simulink model "ThomBBa_Drone"  (R2023a)
settings: Solver=VariableStepAuto  StartTime=0.0  StopTime=10  RelTol=1e-3
values from neighbouring files (symbols this model uses):
  J = [0.00031              0              -0.000004657 ... (first row only)    [paramm.m]
  K = 1256.637    [paramm.m]
  Km = 6.1028207267564559047121275317652e-7    (= 6.10282072676e-07)    [paramm.m]
  Kn = 6.1028207267564559047121275317652e-7    (= 6.10282072676e-07)    [paramm.m]
  l = 0.1125    [paramm.m]
  Phi_air_damping_constant = 0    [paramm.m]
  Psi_air_damping_constant = 0    [paramm.m]
  Tau = 0.001    [paramm.m]
  Theta_air_damping_constant = 0    [paramm.m]
undefined symbols (not defined in the file or in its folder): x_air_damping_ratio, y_air_damping_ratio, z_air_damping_ratio
libraries: dspsigops x15, slpidlib x6
(part 1 of 2)
settings Model: PacingRate=1000  Creator=ThomBBa  LastModifiedBy=ThomBBa
settings DebuggingCC: AlgebraicLoopMsg=none

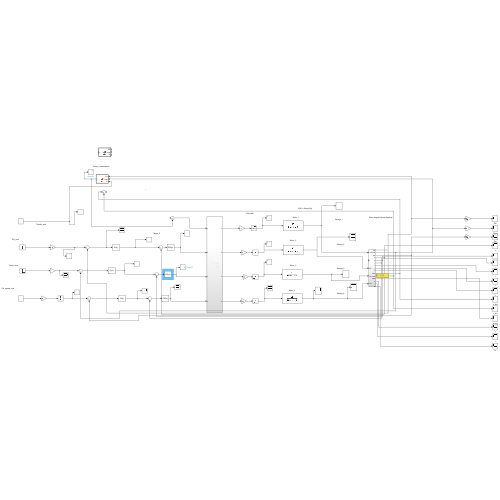
[thumbnail: Simulink's stored preview of the top-level diagram]
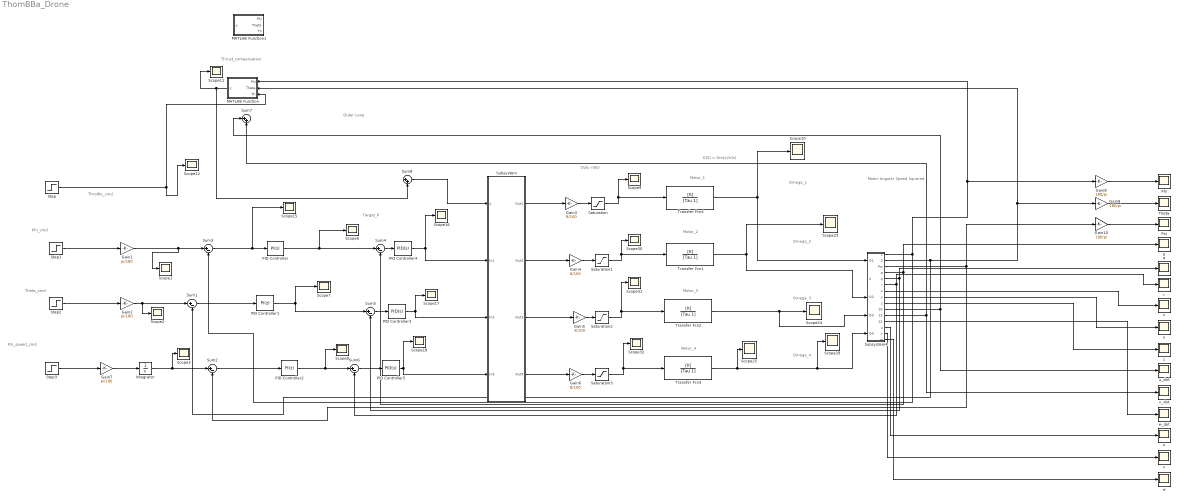
== system ThomBBa_Drone ==
  note: Thrust_compensation
  note: G(S) = Om(s)/V(s)
  note: Omega_1
  note: Motor_1
  note: Motor_2
  note: Omega_2
  note: Throttle_cmd
  note: Target_P
  note: Duty ratio
  note: Motor Angular Speed Squared
  note: Outer Loop
  note: Motor_3
  note: Motor_4
  note: Omega_4
  note: Phi_cmd
  note: Theta_cmd
  note: Psi_speed_cmd
  note: Omega_3
  Gain1 : Gain  Gain=pi/180
  Gain10 : Gain  Gain=180/pi
  Gain2 : Gain  Gain=pi/180
  Gain{3..6} (4 alike) : Gain  Gain=8/100
  Gain7 : Gain  Gain=pi/180
  Gain8 : Gain  Gain=180/pi
  Gain9 : Gain  Gain=180/pi
  Integrator : Integrator
  MATLAB Function : MATLAB Function  TreatAsAtomicUnit=on
  MATLAB Function1 : MATLAB Function  TreatAsAtomicUnit=on
  PID Controller : slpidlib/PID Controller  Controller=PI  Form=Parallel  TimeDomain=Continuous-time  UseExternalTs=off  SampleTime=-1  IntegratorMethod=Forward Euler  FilterMethod=Forward Euler  ControllerParametersSource=internal  P=3  I=0  UseKiTs=off  D=0  N=100  UseFilter=on  TunerSelectOption=Transfer Function Based (PID Tuner App)  InitialConditionSource=internal  InitialConditionForIntegrator=0  InitialConditionForFilter=0  DifferentiatorICPrevScaledInput=0  ExternalReset=none  TrackingMode=off  Kt=1  LimitOutput=off  SatLimitsSource=internal  UpperSaturationLimit=inf  LowerSaturationLimit=-inf  LinearizeAsGain=on  AntiWindupMode=none  Kb=1  LimitIntegrator=off  UpperIntegratorSaturationLimit=inf  LowerIntegratorSaturationLimit=-inf  POutMin=[]  POutMax=[]  IOutMin=[]  IOutMax=[]  DOutMin=[]  DOutMax=[]  NOutMin=[]  NOutMax=[]  SumOutMin=[]  SumOutMax=[]  SaturationOutMin=[]  SaturationOutMax=[]  PParamMin=[]  PParamMax=[]  IParamMin=[]  IParamMax=[]  DParamMin=[]  DParamMax=[]  NParamMin=[]  NParamMax=[]  KbParamMin=[]  KbParamMax=[]  KtParamMin=[]  KtParamMax=[]  KbOutMin=[]  KbOutMax=[]  KtOutMin=[]  KtOutMax=[]  IntegratorOutMin=[]  IntegratorOutMax=[]  FilterOutMin=[]  FilterOutMax=[]  SumI1OutMin=[]  SumI1OutMax=[]  SumI2OutMin=[]  SumI2OutMax=[]  SumI3OutMin=[]  SumI3OutMax=[]  SumI4OutMin=[]  SumI4OutMax=[]  SumDOutMin=[]  SumDOutMax=[]  DifferentiatorOutMin=[]  DifferentiatorOutMax=[]  FilterDiffOutCoefMin=[]  FilterDiffOutCoefMax=[]  ReciprocalOutMin=[]  ReciprocalOutMax=[]  SumDenOutMin=[]  SumDenOutMax=[]  SumNumOutMin=[]  SumNumOutMax=[]  DivideOutMin=[]  DivideOutMax=[]  UdiffTsProdOutMin=[]  UdiffTsProdOutMax=[]  NTsProdOutMin=[]  NTsProdOutMax=[]  UintegralTsProdOutMin=[]  UintegralTsProdOutMax=[]  UngainTsProdOutMin=[]  UngainTsProdOutMax=[]  ClampingZeroOutDataTypeStr=Inherit: Inherit via back propagation  ClampingZeroOutMin=[]  ClampingZeroOutMax=[]  FilterDenConstantOutDataTypeStr=Inherit: Inherit via back propagation  FilterDenConstantOutMin=[]  FilterDenConstantOutMax=[]  PCopyOutDataTypeStr=Inherit: Inherit via back propagation  PCopyOutMin=[]  PCopyOutMax=[]  NCopyOutDataTypeStr=Inherit: Inherit via back propagation  NCopyOutMin=[]  NCopyOutMax=[]  IntegratorContinuousStateAttributes=''  IntegratorStateMustResolveToSignalObject=off  IntegratorRTWStateStorageClass=Auto  FilterContinuousStateAttributes=''  FilterStateMustResolveToSignalObject=off  FilterRTWStateStorageClass=Auto  ParallelPVariant=InternalParameters  IdealPVariant=Disabled  IVariant=InternalParameters  DVariant=Disabled  IntegratorVariant=Continuous  SatVariant=Disabled  AWVariant=Passthrough  PCopyVariant=Disabled  TRVariant=Disabled  FdbkBlocksVariant=Forward  IdealPFdbkVariant=Disabled  SatFdbkVariant=Disabled  DerivativeFilterVariant=Disabled  NVariant=Disabled  NCopyVariant=Disabled_SignalSpec  FilterICVariant=Disabled  IntegratorICVariant=InternalICs  ExternalResetVariant=Disabled  TRSumVariant=Passthrough  SumFdbkVariant=Disabled  SumVariant=Sum_PI  TsampFilterVariant=InternalTs  TsampNgainVariant=Passthrough  TsampIntegralVariant=Disabled_SignalSpec  ExternalSaturationOutDataTypeStr=Inherit: Same as second input
  PID Controller1 : slpidlib/PID Controller  Controller=PI  Form=Parallel  TimeDomain=Discrete-time  UseExternalTs=off  SampleTime=-1  IntegratorMethod=Forward Euler  FilterMethod=Forward Euler  ControllerParametersSource=internal  P=3  I=0  UseKiTs=off  D=0  N=100  UseFilter=on  TunerSelectOption=Transfer Function Based (PID Tuner App)  InitialConditionSource=internal  InitialConditionForIntegrator=0  InitialConditionForFilter=0  DifferentiatorICPrevScaledInput=0  ExternalReset=none  TrackingMode=off  Kt=1  LimitOutput=off  SatLimitsSource=internal  UpperSaturationLimit=inf  LowerSaturationLimit=-inf  LinearizeAsGain=on  AntiWindupMode=none  Kb=1  LimitIntegrator=off  UpperIntegratorSaturationLimit=inf  LowerIntegratorSaturationLimit=-inf  POutMin=[]  POutMax=[]  IOutMin=[]  IOutMax=[]  DOutMin=[]  DOutMax=[]  NOutMin=[]  NOutMax=[]  SumOutMin=[]  SumOutMax=[]  SaturationOutMin=[]  SaturationOutMax=[]  PParamMin=[]  PParamMax=[]  IParamMin=[]  IParamMax=[]  DParamMin=[]  DParamMax=[]  NParamMin=[]  NParamMax=[]  KbParamMin=[]  KbParamMax=[]  KtParamMin=[]  KtParamMax=[]  KbOutMin=[]  KbOutMax=[]  KtOutMin=[]  KtOutMax=[]  IntegratorOutMin=[]  IntegratorOutMax=[]  FilterOutMin=[]  FilterOutMax=[]  SumI1OutMin=[]  SumI1OutMax=[]  SumI2OutMin=[]  SumI2OutMax=[]  SumI3OutMin=[]  SumI3OutMax=[]  SumI4OutMin=[]  SumI4OutMax=[]  SumDOutMin=[]  SumDOutMax=[]  DifferentiatorOutMin=[]  DifferentiatorOutMax=[]  FilterDiffOutCoefMin=[]  FilterDiffOutCoefMax=[]  ReciprocalOutMin=[]  ReciprocalOutMax=[]  SumDenOutMin=[]  SumDenOutMax=[]  SumNumOutMin=[]  SumNumOutMax=[]  DivideOutMin=[]  DivideOutMax=[]  UdiffTsProdOutMin=[]  UdiffTsProdOutMax=[]  NTsProdOutMin=[]  NTsProdOutMax=[]  UintegralTsProdOutMin=[]  UintegralTsProdOutMax=[]  UngainTsProdOutMin=[]  UngainTsProdOutMax=[]  ClampingZeroOutDataTypeStr=Inherit: Inherit via back propagation  ClampingZeroOutMin=[]  ClampingZeroOutMax=[]  FilterDenConstantOutDataTypeStr=Inherit: Inherit via back propagation  FilterDenConstantOutMin=[]  FilterDenConstantOutMax=[]  PCopyOutDataTypeStr=Inherit: Inherit via back propagation  PCopyOutMin=[]  PCopyOutMax=[]  NCopyOutDataTypeStr=Inherit: Inherit via back propagation  NCopyOutMin=[]  NCopyOutMax=[]  IntegratorContinuousStateAttributes=''  IntegratorStateMustResolveToSignalObject=off  IntegratorRTWStateStorageClass=Auto  FilterContinuousStateAttributes=''  FilterStateMustResolveToSignalObject=off  FilterRTWStateStorageClass=Auto  ParallelPVariant=InternalParameters  IdealPVariant=Disabled  IVariant=InternalParameters  DVariant=Disabled  IntegratorVariant=Discrete  SatVariant=Disabled  AWVariant=Passthrough  PCopyVariant=Disabled  TRVariant=Disabled  FdbkBlocksVariant=Forward  IdealPFdbkVariant=Disabled  SatFdbkVariant=Disabled  DerivativeFilterVariant=Disabled  NVariant=Disabled  NCopyVariant=Disabled_SignalSpec  FilterICVariant=Disabled  IntegratorICVariant=InternalICs  ExternalResetVariant=Disabled  TRSumVariant=Passthrough  SumFdbkVariant=Disabled  SumVariant=Sum_PI  TsampFilterVariant=InternalTs  TsampNgainVariant=Passthrough  TsampIntegralVariant=Disabled_SignalSpec  ExternalSaturationOutDataTypeStr=Inherit: Same as second input
  PID Controller2 : slpidlib/PID Controller  Controller=PI  Form=Parallel  TimeDomain=Discrete-time  UseExternalTs=off  SampleTime=-1  IntegratorMethod=Forward Euler  FilterMethod=Forward Euler  ControllerParametersSource=internal  P=1  I=0  UseKiTs=off  D=0  N=100  UseFilter=on  TunerSelectOption=Transfer Function Based (PID Tuner App)  InitialConditionSource=internal  InitialConditionForIntegrator=0  InitialConditionForFilter=0  DifferentiatorICPrevScaledInput=0  ExternalReset=none  TrackingMode=off  Kt=1  LimitOutput=off  SatLimitsSource=internal  UpperSaturationLimit=inf  LowerSaturationLimit=-inf  LinearizeAsGain=on  AntiWindupMode=none  Kb=1  LimitIntegrator=off  UpperIntegratorSaturationLimit=inf  LowerIntegratorSaturationLimit=-inf  POutMin=[]  POutMax=[]  IOutMin=[]  IOutMax=[]  DOutMin=[]  DOutMax=[]  NOutMin=[]  NOutMax=[]  SumOutMin=[]  SumOutMax=[]  SaturationOutMin=[]  SaturationOutMax=[]  PParamMin=[]  PParamMax=[]  IParamMin=[]  IParamMax=[]  DParamMin=[]  DParamMax=[]  NParamMin=[]  NParamMax=[]  KbParamMin=[]  KbParamMax=[]  KtParamMin=[]  KtParamMax=[]  KbOutMin=[]  KbOutMax=[]  KtOutMin=[]  KtOutMax=[]  IntegratorOutMin=[]  IntegratorOutMax=[]  FilterOutMin=[]  FilterOutMax=[]  SumI1OutMin=[]  SumI1OutMax=[]  SumI2OutMin=[]  SumI2OutMax=[]  SumI3OutMin=[]  SumI3OutMax=[]  SumI4OutMin=[]  SumI4OutMax=[]  SumDOutMin=[]  SumDOutMax=[]  DifferentiatorOutMin=[]  DifferentiatorOutMax=[]  FilterDiffOutCoefMin=[]  FilterDiffOutCoefMax=[]  ReciprocalOutMin=[]  ReciprocalOutMax=[]  SumDenOutMin=[]  SumDenOutMax=[]  SumNumOutMin=[]  SumNumOutMax=[]  DivideOutMin=[]  DivideOutMax=[]  UdiffTsProdOutMin=[]  UdiffTsProdOutMax=[]  NTsProdOutMin=[]  NTsProdOutMax=[]  UintegralTsProdOutMin=[]  UintegralTsProdOutMax=[]  UngainTsProdOutMin=[]  UngainTsProdOutMax=[]  ClampingZeroOutDataTypeStr=Inherit: Inherit via back propagation  ClampingZeroOutMin=[]  ClampingZeroOutMax=[]  FilterDenConstantOutDataTypeStr=Inherit: Inherit via back propagation  FilterDenConstantOutMin=[]  FilterDenConstantOutMax=[]  PCopyOutDataTypeStr=Inherit: Inherit via back propagation  PCopyOutMin=[]  PCopyOutMax=[]  NCopyOutDataTypeStr=Inherit: Inherit via back propagation  NCopyOutMin=[]  NCopyOutMax=[]  IntegratorContinuousStateAttributes=''  IntegratorStateMustResolveToSignalObject=off  IntegratorRTWStateStorageClass=Auto  FilterContinuousStateAttributes=''  FilterStateMustResolveToSignalObject=off  FilterRTWStateStorageClass=Auto  ParallelPVariant=InternalParameters  IdealPVariant=Disabled  IVariant=InternalParameters  DVariant=Disabled  IntegratorVariant=Discrete  SatVariant=Disabled  AWVariant=Passthrough  PCopyVariant=Disabled  TRVariant=Disabled  FdbkBlocksVariant=Forward  IdealPFdbkVariant=Disabled  SatFdbkVariant=Disabled  DerivativeFilterVariant=Disabled  NVariant=Disabled  NCopyVariant=Disabled_SignalSpec  FilterICVariant=Disabled  IntegratorICVariant=InternalICs  ExternalResetVariant=Disabled  TRSumVariant=Passthrough  SumFdbkVariant=Disabled  SumVariant=Sum_PI  TsampFilterVariant=InternalTs  TsampNgainVariant=Passthrough  TsampIntegralVariant=Disabled_SignalSpec  ExternalSaturationOutDataTypeStr=Inherit: Same as second input
  PID Controller3 : slpidlib/PID Controller  Controller=PID  Form=Parallel  TimeDomain=Continuous-time  UseExternalTs=off  SampleTime=-1  IntegratorMethod=Forward Euler  FilterMethod=Forward Euler  ControllerParametersSource=internal  P=15  I=0  UseKiTs=off  D=3  N=100  UseFilter=on  TunerSelectOption=Transfer Function Based (PID Tuner App)  InitialConditionSource=internal  InitialConditionForIntegrator=0  InitialConditionForFilter=0  DifferentiatorICPrevScaledInput=0  ExternalReset=none  TrackingMode=off  Kt=1  LimitOutput=off  SatLimitsSource=internal  UpperSaturationLimit=inf  LowerSaturationLimit=-inf  LinearizeAsGain=on  AntiWindupMode=none  Kb=1  LimitIntegrator=off  UpperIntegratorSaturationLimit=inf  LowerIntegratorSaturationLimit=-inf  POutMin=[]  POutMax=[]  IOutMin=[]  IOutMax=[]  DOutMin=[]  DOutMax=[]  NOutMin=[]  NOutMax=[]  SumOutMin=[]  SumOutMax=[]  SaturationOutMin=[]  SaturationOutMax=[]  PParamMin=[]  PParamMax=[]  IParamMin=[]  IParamMax=[]  DParamMin=[]  DParamMax=[]  NParamMin=[]  NParamMax=[]  KbParamMin=[]  KbParamMax=[]  KtParamMin=[]  KtParamMax=[]  KbOutMin=[]  KbOutMax=[]  KtOutMin=[]  KtOutMax=[]  IntegratorOutMin=[]  IntegratorOutMax=[]  FilterOutMin=[]  FilterOutMax=[]  SumI1OutMin=[]  SumI1OutMax=[]  SumI2OutMin=[]  SumI2OutMax=[]  SumI3OutMin=[]  SumI3OutMax=[]  SumI4OutMin=[]  SumI4OutMax=[]  SumDOutMin=[]  SumDOutMax=[]  DifferentiatorOutMin=[]  DifferentiatorOutMax=[]  FilterDiffOutCoefMin=[]  FilterDiffOutCoefMax=[]  ReciprocalOutMin=[]  ReciprocalOutMax=[]  SumDenOutMin=[]  SumDenOutMax=[]  SumNumOutMin=[]  SumNumOutMax=[]  DivideOutMin=[]  DivideOutMax=[]  UdiffTsProdOutMin=[]  UdiffTsProdOutMax=[]  NTsProdOutMin=[]  NTsProdOutMax=[]  UintegralTsProdOutMin=[]  UintegralTsProdOutMax=[]  UngainTsProdOutMin=[]  UngainTsProdOutMax=[]  ClampingZeroOutDataTypeStr=Inherit: Inherit via back propagation  ClampingZeroOutMin=[]  ClampingZeroOutMax=[]  FilterDenConstantOutDataTypeStr=Inherit: Inherit via back propagation  FilterDenConstantOutMin=[]  FilterDenConstantOutMax=[]  PCopyOutDataTypeStr=Inherit: Inherit via back propagation  PCopyOutMin=[]  PCopyOutMax=[]  NCopyOutDataTypeStr=Inherit: Inherit via back propagation  NCopyOutMin=[]  NCopyOutMax=[]  IntegratorContinuousStateAttributes=''  IntegratorStateMustResolveToSignalObject=off  IntegratorRTWStateStorageClass=Auto  FilterContinuousStateAttributes=''  FilterStateMustResolveToSignalObject=off  FilterRTWStateStorageClass=Auto  ParallelPVariant=InternalParameters  IdealPVariant=Disabled  IVariant=InternalParameters  DVariant=InternalParameters  IntegratorVariant=Continuous  SatVariant=Disabled  AWVariant=Passthrough  PCopyVariant=Disabled  TRVariant=Disabled  FdbkBlocksVariant=Forward  IdealPFdbkVariant=Disabled  SatFdbkVariant=Disabled  DerivativeFilterVariant=ContFilter  NVariant=InternalParameters  NCopyVariant=Disabled  FilterICVariant=InternalICsFilter  IntegratorICVariant=InternalICs  ExternalResetVariant=Disabled  TRSumVariant=Passthrough  SumFdbkVariant=Disabled  SumVariant=Sum_PID  TsampFilterVariant=InternalTs  TsampNgainVariant=Passthrough  TsampIntegralVariant=Disabled_SignalSpec  ExternalSaturationOutDataTypeStr=Inherit: Same as second input
  PID Controller4 : slpidlib/PID Controller  Controller=PID  Form=Parallel  TimeDomain=Continuous-time  UseExternalTs=off  SampleTime=-1  IntegratorMethod=Forward Euler  FilterMethod=Forward Euler  ControllerParametersSource=internal  P=10  I=0  UseKiTs=off  D=3  N=100  UseFilter=on  TunerSelectOption=Transfer Function Based (PID Tuner App)  InitialConditionSource=internal  InitialConditionForIntegrator=0  InitialConditionForFilter=0  DifferentiatorICPrevScaledInput=0  ExternalReset=none  TrackingMode=off  Kt=1  LimitOutput=off  SatLimitsSource=internal  UpperSaturationLimit=inf  LowerSaturationLimit=-inf  LinearizeAsGain=on  AntiWindupMode=none  Kb=1  LimitIntegrator=off  UpperIntegratorSaturationLimit=inf  LowerIntegratorSaturationLimit=-inf  POutMin=[]  POutMax=[]  IOutMin=[]  IOutMax=[]  DOutMin=[]  DOutMax=[]  NOutMin=[]  NOutMax=[]  SumOutMin=[]  SumOutMax=[]  SaturationOutMin=[]  SaturationOutMax=[]  PParamMin=[]  PParamMax=[]  IParamMin=[]  IParamMax=[]  DParamMin=[]  DParamMax=[]  NParamMin=[]  NParamMax=[]  KbParamMin=[]  KbParamMax=[]  KtParamMin=[]  KtParamMax=[]  KbOutMin=[]  KbOutMax=[]  KtOutMin=[]  KtOutMax=[]  IntegratorOutMin=[]  IntegratorOutMax=[]  FilterOutMin=[]  FilterOutMax=[]  SumI1OutMin=[]  SumI1OutMax=[]  SumI2OutMin=[]  SumI2OutMax=[]  SumI3OutMin=[]  SumI3OutMax=[]  SumI4OutMin=[]  SumI4OutMax=[]  SumDOutMin=[]  SumDOutMax=[]  DifferentiatorOutMin=[]  DifferentiatorOutMax=[]  FilterDiffOutCoefMin=[]  FilterDiffOutCoefMax=[]  ReciprocalOutMin=[]  ReciprocalOutMax=[]  SumDenOutMin=[]  SumDenOutMax=[]  SumNumOutMin=[]  SumNumOutMax=[]  DivideOutMin=[]  DivideOutMax=[]  UdiffTsProdOutMin=[]  UdiffTsProdOutMax=[]  NTsProdOutMin=[]  NTsProdOutMax=[]  UintegralTsProdOutMin=[]  UintegralTsProdOutMax=[]  UngainTsProdOutMin=[]  UngainTsProdOutMax=[]  ClampingZeroOutDataTypeStr=Inherit: Inherit via back propagation  ClampingZeroOutMin=[]  ClampingZeroOutMax=[]  FilterDenConstantOutDataTypeStr=Inherit: Inherit via back propagation  FilterDenConstantOutMin=[]  FilterDenConstantOutMax=[]  PCopyOutDataTypeStr=Inherit: Inherit via back propagation  PCopyOutMin=[]  PCopyOutMax=[]  NCopyOutDataTypeStr=Inherit: Inherit via back propagation  NCopyOutMin=[]  NCopyOutMax=[]  IntegratorContinuousStateAttributes=''  IntegratorStateMustResolveToSignalObject=off  IntegratorRTWStateStorageClass=Auto  FilterContinuousStateAttributes=''  FilterStateMustResolveToSignalObject=off  FilterRTWStateStorageClass=Auto  ParallelPVariant=InternalParameters  IdealPVariant=Disabled  IVariant=InternalParameters  DVariant=InternalParameters  IntegratorVariant=Continuous  SatVariant=Disabled  AWVariant=Passthrough  PCopyVariant=Disabled  TRVariant=Disabled  FdbkBlocksVariant=Forward  IdealPFdbkVariant=Disabled  SatFdbkVariant=Disabled  DerivativeFilterVariant=ContFilter  NVariant=InternalParameters  NCopyVariant=Disabled  FilterICVariant=InternalICsFilter  IntegratorICVariant=InternalICs  ExternalResetVariant=Disabled  TRSumVariant=Passthrough  SumFdbkVariant=Disabled  SumVariant=Sum_PID  TsampFilterVariant=InternalTs  TsampNgainVariant=Passthrough  TsampIntegralVariant=Disabled_SignalSpec  ExternalSaturationOutDataTypeStr=Inherit: Same as second input
  PID Controller5 : slpidlib/PID Controller  Controller=PID  Form=Parallel  TimeDomain=Continuous-time  UseExternalTs=off  SampleTime=-1  IntegratorMethod=Forward Euler  FilterMethod=Forward Euler  ControllerParametersSource=internal  P=3  I=0  UseKiTs=off  D=0  N=100  UseFilter=on  TunerSelectOption=Transfer Function Based (PID Tuner App)  InitialConditionSource=internal  InitialConditionForIntegrator=0  InitialConditionForFilter=0  DifferentiatorICPrevScaledInput=0  ExternalReset=none  TrackingMode=off  Kt=1  LimitOutput=off  SatLimitsSource=internal  UpperSaturationLimit=inf  LowerSaturationLimit=-inf  LinearizeAsGain=on  AntiWindupMode=none  Kb=1  LimitIntegrator=off  UpperIntegratorSaturationLimit=inf  LowerIntegratorSaturationLimit=-inf  POutMin=[]  POutMax=[]  IOutMin=[]  IOutMax=[]  DOutMin=[]  DOutMax=[]  NOutMin=[]  NOutMax=[]  SumOutMin=[]  SumOutMax=[]  SaturationOutMin=[]  SaturationOutMax=[]  PParamMin=[]  PParamMax=[]  IParamMin=[]  IParamMax=[]  DParamMin=[]  DParamMax=[]  NParamMin=[]  NParamMax=[]  KbParamMin=[]  KbParamMax=[]  KtParamMin=[]  KtParamMax=[]  KbOutMin=[]  KbOutMax=[]  KtOutMin=[]  KtOutMax=[]  IntegratorOutMin=[]  IntegratorOutMax=[]  FilterOutMin=[]  FilterOutMax=[]  SumI1OutMin=[]  SumI1OutMax=[]  SumI2OutMin=[]  SumI2OutMax=[]  SumI3OutMin=[]  SumI3OutMax=[]  SumI4OutMin=[]  SumI4OutMax=[]  SumDOutMin=[]  SumDOutMax=[]  DifferentiatorOutMin=[]  DifferentiatorOutMax=[]  FilterDiffOutCoefMin=[]  FilterDiffOutCoefMax=[]  ReciprocalOutMin=[]  ReciprocalOutMax=[]  SumDenOutMin=[]  SumDenOutMax=[]  SumNumOutMin=[]  SumNumOutMax=[]  DivideOutMin=[]  DivideOutMax=[]  UdiffTsProdOutMin=[]  UdiffTsProdOutMax=[]  NTsProdOutMin=[]  NTsProdOutMax=[]  UintegralTsProdOutMin=[]  UintegralTsProdOutMax=[]  UngainTsProdOutMin=[]  UngainTsProdOutMax=[]  ClampingZeroOutDataTypeStr=Inherit: Inherit via back propagation  ClampingZeroOutMin=[]  ClampingZeroOutMax=[]  FilterDenConstantOutDataTypeStr=Inherit: Inherit via back propagation  FilterDenConstantOutMin=[]  FilterDenConstantOutMax=[]  PCopyOutDataTypeStr=Inherit: Inherit via back propagation  PCopyOutMin=[]  PCopyOutMax=[]  NCopyOutDataTypeStr=Inherit: Inherit via back propagation  NCopyOutMin=[]  NCopyOutMax=[]  IntegratorContinuousStateAttributes=''  IntegratorStateMustResolveToSignalObject=off  IntegratorRTWStateStorageClass=Auto  FilterContinuousStateAttributes=''  FilterStateMustResolveToSignalObject=off  FilterRTWStateStorageClass=Auto  ParallelPVariant=InternalParameters  IdealPVariant=Disabled  IVariant=InternalParameters  DVariant=InternalParameters  IntegratorVariant=Continuous  SatVariant=Disabled  AWVariant=Passthrough  PCopyVariant=Disabled  TRVariant=Disabled  FdbkBlocksVariant=Forward  IdealPFdbkVariant=Disabled  SatFdbkVariant=Disabled  DerivativeFilterVariant=ContFilter  NVariant=InternalParameters  NCopyVariant=Disabled  FilterICVariant=InternalICsFilter  IntegratorICVariant=InternalICs  ExternalResetVariant=Disabled  TRSumVariant=Passthrough  SumFdbkVariant=Disabled  SumVariant=Sum_PID  TsampFilterVariant=InternalTs  TsampNgainVariant=Passthrough  TsampIntegralVariant=Disabled_SignalSpec  ExternalSaturationOutDataTypeStr=Inherit: Same as second input
  Phi : Scope
  Psi : Scope
  Saturation{,1..3} (4 alike) : Saturate  UpperLimit=8.4  LowerLimit=0
  Scope{1..3,6..12,15..18,23..25,29..32} (21 alike) : Scope
  Step : Step  Time=0  Before=19.933  After=19.933  SampleTime=0
  Step1 : Step  Time=2  After=5  SampleTime=0
  Step2 : Step  Time=2  After=-10  SampleTime=0
  Step3 : Step  After=0  SampleTime=0
  Subsystem : Subsystem
  Subsystem4 : Subsystem
  Sum{1..6} (6 alike) : Sum  Inputs=|+-
  Sum7 : Sum  Inputs=|++
  Sum8 : Sum  Inputs=|++
  Theta : Scope
  Transfer Fcn1 : TransferFcn  Numerator=[K]  Denominator=[Tau 1]
  Transfer Fcn2 : TransferFcn  Numerator=[K]  Denominator=[Tau 1]
  Transfer Fcn3 : TransferFcn  Numerator=[K]  Denominator=[Tau 1]
  Transfer Fcn4 : TransferFcn  Numerator=[K]  Denominator=[Tau 1]  ParameterTunability=Optimized
  p : Scope
  q : Scope
  r : Scope
  u : Scope
  u_dot : Scope
  v : Scope
  v_dot : Scope
  w : Scope
  w_dot : Scope
  x : Scope
  y : Scope
  z : Scope
  wires:
  Gain4/1 -> Saturation1/1
  Gain3/1 -> Saturation/1
  Gain5/1 -> Saturation2/1
  Gain6/1 -> Saturation3/1
  Step2/1 -> Gain2/1
  Step3/1 -> Gain7/1
  Step1/1 -> Gain1/1
  Transfer Fcn1/1 -> Subsystem4/3(O2), Scope23/1
  Transfer Fcn3/1 -> Subsystem4/5(O4), Scope29/1, Scope25/1
  Transfer Fcn2/1 -> Subsystem4/4(O3), Scope24/1
  Transfer Fcn4/1 -> Subsystem4/1(O1), Scope10/1
  Subsystem4/2(Theta) -> Sum1/2, MATLAB Function/2(Theta), Gain9/1
  Subsystem4/3(Psi) -> Sum2/2, Gain10/1
  Gain1/1 -> Sum3/1, Scope1/1
  Gain7/1 -> Integrator/1
  Gain2/1 -> Sum1/1, Scope2/1
  Sum3/1 -> Scope15/1, PID Controller/1
  PID Controller/1 -> Scope6/1, Sum4/1
  PID Controller1/1 -> Sum5/1, Scope7/1
  PID Controller2/1 -> Sum6/1, Scope8/1
  Sum1/1 -> PID Controller1/1
  Sum2/1 -> PID Controller2/1
  Subsystem4/1(Phi) -> MATLAB Function/1(Phi), Gain8/1, Sum3/2
  Sum4/1 -> PID Controller4/1
  Subsystem4/4(p) -> p/1, Sum4/2
  PID Controller4/1 -> Subsystem/2(In1), Scope16/1
  Gain8/1 -> Phi/1
  PID Controller3/1 -> Subsystem/3(In2), Scope17/1
  PID Controller5/1 -> Scope18/1, Subsystem/4(In3)
  Sum6/1 -> PID Controller5/1
  Sum5/1 -> PID Controller3/1
  Subsystem4/5(q) -> q/1, Sum5/2
  Subsystem4/6(r) -> r/1, Sum6/2
  Gain9/1 -> Theta/1
  Gain10/1 -> Psi/1
  Subsystem/1(Out1) -> Gain3/1
  Subsystem/2(Out2) -> Gain4/1
  Subsystem/4(Out4) -> Gain6/1
  Subsystem/3(Out3) -> Gain5/1
  Saturation/1 -> Transfer Fcn4/1, Scope9/1
  Saturation1/1 -> Scope30/1, Transfer Fcn1/1
  Saturation2/1 -> Scope31/1, Transfer Fcn2/1
  Saturation3/1 -> Scope32/1, Transfer Fcn3/1
  Integrator/1 -> Scope3/1, Sum2/1
  Step/1 -> Scope12/1, MATLAB Function/3(Th)
  MATLAB Function/1(y) -> Sum8/2, Scope11/1
  Subsystem4/7(x) -> x/1
  Subsystem4/8(y) -> y/1
  Subsystem4/9(z) -> z/1
  Subsystem4/10(udot) -> Sum7/1, u_dot/1
  Subsystem4/11(vdot) -> Sum7/2, v_dot/1
  Sum8/1 -> Subsystem/1(y)
  Subsystem4/12(wdot) -> w_dot/1
  Subsystem4/13(u) -> u/1
  Subsystem4/14(v) -> v/1
  Subsystem4/15(w) -> w/1

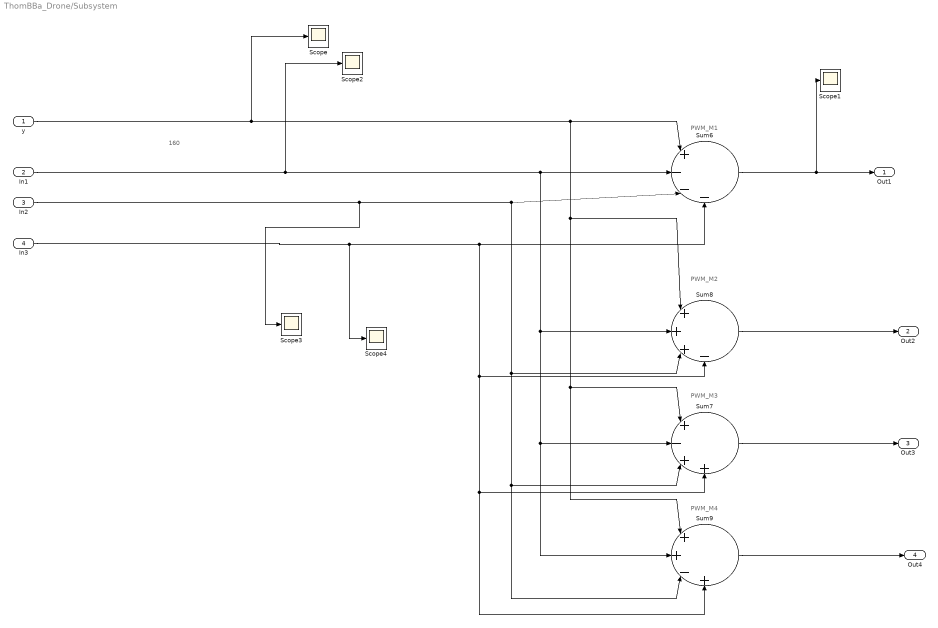
== system ThomBBa_Drone/Subsystem ==
  note: 160
  note: PWM_M4
  note: PWM_M3
  note: PWM_M2
  note: PWM_M1
  y : Inport
  In1 : Inport  Port=2
  In2 : Inport  Port=3
  In3 : Inport  Port=4
  Scope{,1..4} (5 alike) : Scope
  Sum6 : Sum  Inputs=|+---
  Sum7 : Sum  Inputs=|+-++
  Sum8 : Sum  Inputs=|+++-
  Sum9 : Sum  Inputs=|++-+
  Out1 : Outport
  Out2 : Outport  Port=2
  Out3 : Outport  Port=3
  Out4 : Outport  Port=4
  wires:
  y/1 -> Scope/1, Sum6/1, Sum8/1, Sum9/1, Sum7/1
  Sum6/1 -> Out1/1, Scope1/1
  Sum8/1 -> Out2/1
  Sum7/1 -> Out3/1
  Sum9/1 -> Out4/1
  In1/1 -> Scope2/1, Sum6/2, Sum8/2, Sum9/2, Sum7/2
  In2/1 -> Scope3/1, Sum9/3, Sum7/3, Sum8/3, Sum6/3
  In3/1 -> Sum6/4, Sum9/4, Sum7/4, Sum8/4, Scope4/1

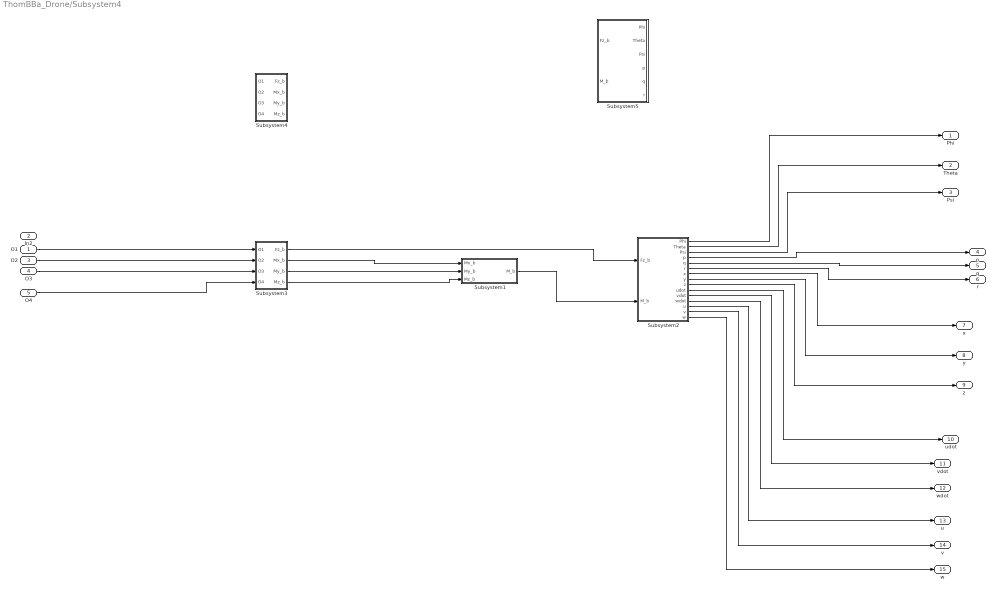
== system ThomBBa_Drone/Subsystem4 ==
  O1 : Inport
  In2 : Inport  Port=2
  O2 : Inport  Port=3
  O3 : Inport  Port=4
  O4 : Inport  Port=5
  Subsystem1 : Subsystem
  Subsystem2 : Subsystem
  Subsystem3 : Subsystem
  Subsystem4 : Subsystem
  Subsystem5 : Subsystem
  Phi : Outport
  Theta : Outport  Port=2
  Psi : Outport  Port=3
  p : Outport  Port=4
  q : Outport  Port=5
  r : Outport  Port=6
  x : Outport  Port=7
  y : Outport  Port=8
  z : Outport  Port=9
  udot : Outport  Port=10
  vdot : Outport  Port=11
  wdot : Outport  Port=12
  u : Outport  Port=13
  v : Outport  Port=14
  w : Outport  Port=15
  wires:
  O2/1 -> Subsystem3/2(O2)
  Subsystem2/5(q) -> q/1
  Subsystem2/6(r) -> r/1
  O1/1 -> Subsystem3/1(O1)
  O3/1 -> Subsystem3/3(O3)
  O4/1 -> Subsystem3/4(O4)
  Subsystem2/4(p) -> p/1
  Subsystem1/1(M_b) -> Subsystem2/2(M_b)
  Subsystem3/2(Mx_b) -> Subsystem1/1(Mx_b)
  Subsystem3/3(My_b) -> Subsystem1/2(My_b)
  Subsystem3/4(Mz_b) -> Subsystem1/3(Mz_b)
  Subsystem3/1(Fz_b) -> Subsystem2/1(Fz_b)
  Subsystem2/1(Phi) -> Phi/1
  Subsystem2/2(Theta) -> Theta/1
  Subsystem2/3(Psi) -> Psi/1
  Subsystem2/7(x) -> x/1
  Subsystem2/8(y) -> y/1
  Subsystem2/9(z) -> z/1
  Subsystem2/10(udot) -> udot/1
  Subsystem2/11(vdot) -> vdot/1
  Subsystem2/12(wdot) -> wdot/1
  Subsystem2/13(u) -> u/1
  Subsystem2/14(v) -> v/1
  Subsystem2/15(w) -> w/1

== system ThomBBa_Drone/Subsystem4/Subsystem1 ==
  Mx_b : Inport
  My_b : Inport  Port=2
  Mz_b : Inport  Port=3
  MATLAB Function1 : MATLAB Function  TreatAsAtomicUnit=on
  M_b : Outport
  wires:
  MATLAB Function1/1(M) -> M_b/1
  Mx_b/1 -> MATLAB Function1/1(Mx)
  My_b/1 -> MATLAB Function1/2(My)
  Mz_b/1 -> MATLAB Function1/3(Mz)

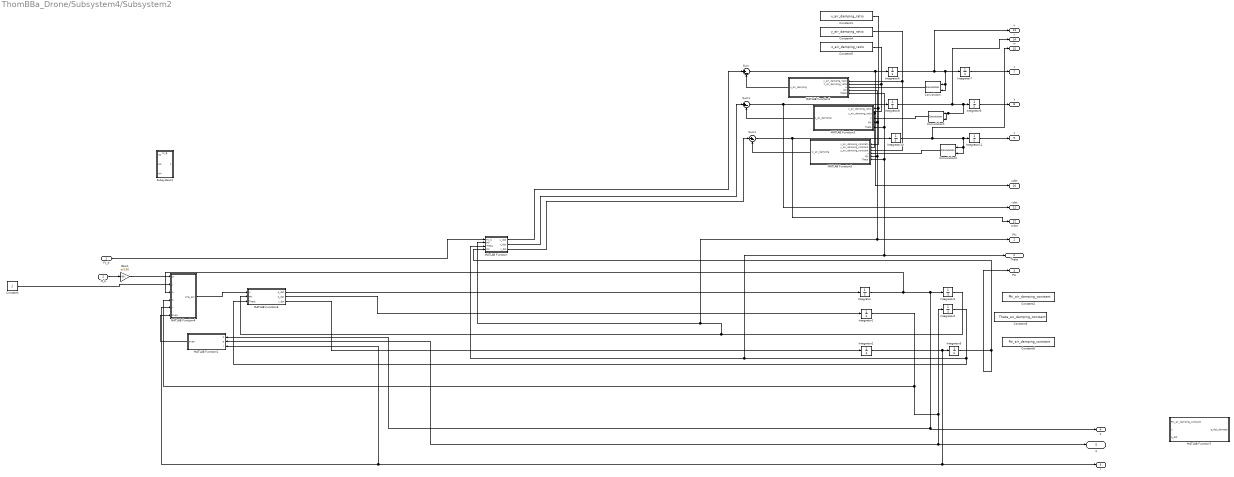
== system ThomBBa_Drone/Subsystem4/Subsystem2 ==
  Fz_b : Inport
  M_b : Inport  Port=2
  Constant : Constant  Value=J
  Constant1 : Constant  Value=x_air_damping_ratio
  Constant2 : Constant  Value=Phi_air_damping_constant
  Constant3 : Constant  Value=Theta_air_damping_constant
  Constant4 : Constant  Value=y_air_damping_ratio
  Constant5 : Constant  Value=z_air_damping_ratio
  Constant6 : Constant  Value=Psi_air_damping_constant
  Convolution : dspsigops/Convolution  domain=Time  roundingMode=Floor  overflowMode=off  outputDataTypeStr=Inherit: Same as accumulator  outputMin=[]  outputMax=[]  outputLastDataTypeStr=Inherit: Same as accumulator
  Convolution1 : dspsigops/Convolution  domain=Time  roundingMode=Floor  overflowMode=off  outputDataTypeStr=Inherit: Same as accumulator  outputMin=[]  outputMax=[]  outputLastDataTypeStr=Inherit: Same as accumulator
  Convolution2 : dspsigops/Convolution  domain=Time  roundingMode=Floor  overflowMode=off  outputDataTypeStr=Inherit: Same as accumulator  outputMin=[]  outputMax=[]  outputLastDataTypeStr=Inherit: Same as accumulator
  Gain1 : Gain  Gain=pi/180
  Integrator{,1..11} (12 alike) : Integrator
  MATLAB Function : MATLAB Function  TreatAsAtomicUnit=on
  MATLAB Function1 : MATLAB Function  TreatAsAtomicUnit=on
  MATLAB Function2 : MATLAB Function  TreatAsAtomicUnit=on
  MATLAB Function3 : MATLAB Function  TreatAsAtomicUnit=on
  MATLAB Function4 : MATLAB Function  TreatAsAtomicUnit=on
  MATLAB Function5 : MATLAB Function  TreatAsAtomicUnit=on
  MATLAB Function6 : MATLAB Function  TreatAsAtomicUnit=on
  MATLAB Function7 : MATLAB Function  TreatAsAtomicUnit=on
  Subsystem2 : Subsystem
      settings: PortSchema="{\"entries\":[{\"content\":{\"sides\":[{\"content\":{\"connectorIds\":[\"In1\",\"In2\",\"In3\"]},\"type\":\"ConnectorPlacement.EquallySpacedRectSide\",\"uuid\":\"7e47c556-e7ea-4b92-bd73-2618c8afdf66\"},{\"content\":{\"connectorIds\":[\"Out1\"],\"side\":\"RIGHT\"},\"type\":\"ConnectorPlacement.EquallySpacedRectSide\",\"uuid\":\"8df0990a-ca25-4c34-ba36-930149f0a751\"},{\"content\":{\"connectorIds\":[\"In4\"],\"side\":\"TOP\"},\"type\":\"ConnectorPlacement.EquallySpacedRectSide\",\"uuid\":\"95f61e22-0c49-4373-add7-f41402ac3268\"},{\"content\":{\"side\":\"BOTTOM\"},\"type\":\"ConnectorPlacement.EquallySpacedRectSide\",\"uuid\":\"d89dd497-fba1-4e7c-8f58-49be8a5c83fa\"}]},\"type\":\"ConnectorPlacement.EquallySpacedConnector\",\"uuid\":\"f38f0594-1519-401a-85c8-093cd101747f\"}],\"packageUris\":[\"http://schema.mathworks.com/mf0/Connector/R2020b\"],\"version\":\"1.0\"}"
  Sum : Sum  Inputs=|+-
  Sum1 : Sum  Inputs=|+-
  Sum2 : Sum  Inputs=|+-
  Phi : Outport
  Theta : Outport  Port=2
  Psi : Outport  Port=3
  p : Outport  Port=4
  q : Outport  Port=5
  r : Outport  Port=6
  x : Outport  Port=7
  y : Outport  Port=8
  z : Outport  Port=9
  udot : Outport  Port=10
  vdot : Outport  Port=11
  wdot : Outport  Port=12
  u : Outport  Port=13
  v : Outport  Port=14
  w : Outport  Port=15
  wires:
  M_b/1 -> Gain1/1
  Integrator/1 -> MATLAB Function1/1(p), p/1, Integrator3/1, MATLAB Function4/3(p)
  Fz_b/1 -> MATLAB Function/1(Fz_b)
  MATLAB Function/3(r_dot) -> Sum2/1
  MATLAB Function4/1(Ang_acc) -> MATLAB Function6/1(u)
  Gain1/1 -> MATLAB Function4/1(M)
  Integrator3/1 -> MATLAB Function5/5(Phi), MATLAB Function2/4(Phi), MATLAB Function3/4(Phi), Phi/1, MATLAB Function/2(Phi), MATLAB Function6/2(Phi)
  Integrator4/1 -> MATLAB Function6/3(Theta), MATLAB Function5/6(Theta), MATLAB Function2/5(Theta), MATLAB Function3/5(Theta), Theta/1, MATLAB Function/3(Theta)
  Integrator5/1 -> Psi/1, MATLAB Function/4(Psi)
  MATLAB Function1/1(skew) -> MATLAB Function4/6(skew)
  Constant/1 -> MATLAB Function4/2(J)
  Integrator6/1 -> u/1, Convolution/2, Convolution/1, Integrator7/1
  Integrator7/1 -> x/1
  Integrator9/1 -> y/1
  Integrator11/1 -> z/1
  Sum/1 -> udot/1, Integrator6/1
  Integrator8/1 -> v/1, Convolution1/2, Convolution1/1, Integrator9/1
  Sum1/1 -> vdot/1, Integrator8/1
  Integrator10/1 -> w/1, Convolution2/2, Convolution2/1, Integrator11/1
  MATLAB Function5/1(w_air_damping) -> Sum2/2
  Sum2/1 -> Integrator10/1, wdot/1
  Convolution/1 -> MATLAB Function2/3(u)
  Convolution1/1 -> MATLAB Function3/3(u)
  Convolution2/1 -> MATLAB Function5/4(u)
  MATLAB Function6/2(q_dot) -> Integrator1/1
  Integrator1/1 -> MATLAB Function1/2(q), q/1, Integrator4/1, MATLAB Function4/4(q)
  Integrator2/1 -> MATLAB Function4/5(r), MATLAB Function1/3(r), r/1, Integrator5/1
  MATLAB Function6/3(r_dot) -> Integrator2/1
  MATLAB Function/1(u_dot) -> Sum/1
  MATLAB Function/2(v_dot) -> Sum1/1
  MATLAB Function2/1(u_air_damping) -> Sum/2
  MATLAB Function3/1(u_air_damping) -> Sum1/2
  Constant4/1 -> MATLAB Function5/3(z_air_damping_constant), MATLAB Function2/1(x_air_damping_ratio)
  Constant5/1 -> MATLAB Function5/2(y_air_damping_constant), MATLAB Function3/2(z_air_damping_ratio), MATLAB Function2/2(z_air_damping_ratio)
  Constant1/1 -> MATLAB Function5/1(x_air_damping_constatn), MATLAB Function3/1(x_air_damping_ratio)
  MATLAB Function6/1(p_dot) -> Integrator/1

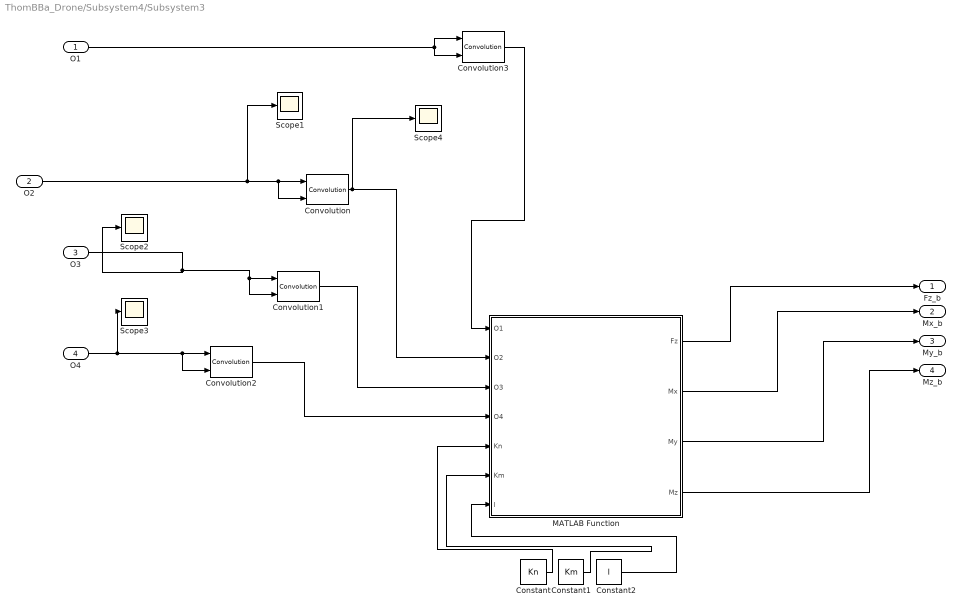
== system ThomBBa_Drone/Subsystem4/Subsystem3 ==
  O1 : Inport
  O2 : Inport  Port=2
  O3 : Inport  Port=3
  O4 : Inport  Port=4
  Constant : Constant  Value=Kn
  Constant1 : Constant  Value=Km
  Constant2 : Constant  Value=l
  Convolution{,1..3} (4 alike) : dspsigops/Convolution  domain=Time  roundingMode=Floor  overflowMode=off  outputDataTypeStr=Inherit: Same as accumulator  outputMin=[]  outputMax=[]  outputLastDataTypeStr=Inherit: Same as accumulator
  MATLAB Function : MATLAB Function  TreatAsAtomicUnit=on
  Scope{1..4} (4 alike) : Scope
  Fz_b : Outport
  Mx_b : Outport  Port=2
  My_b : Outport  Port=3
  Mz_b : Outport  Port=4
  wires:
  MATLAB Function/1(Fz) -> Fz_b/1
  MATLAB Function/3(My) -> My_b/1
  MATLAB Function/4(Mz) -> Mz_b/1
  MATLAB Function/2(Mx) -> Mx_b/1
  Constant/1 -> MATLAB Function/5(Kn)
  Constant1/1 -> MATLAB Function/6(Km)
  Constant2/1 -> MATLAB Function/7(l)
  O2/1 -> Convolution/2, Convolution/1, Scope1/1
  O3/1 -> Convolution1/2, Convolution1/1, Scope2/1
  Convolution1/1 -> MATLAB Function/3(O3)
  O4/1 -> Convolution2/2, Convolution2/1, Scope3/1
  Convolution2/1 -> MATLAB Function/4(O4)
  O1/1 -> Convolution3/1, Convolution3/2
  Convolution3/1 -> MATLAB Function/1(O1)
  Convolution/1 -> Scope4/1, MATLAB Function/2(O2)

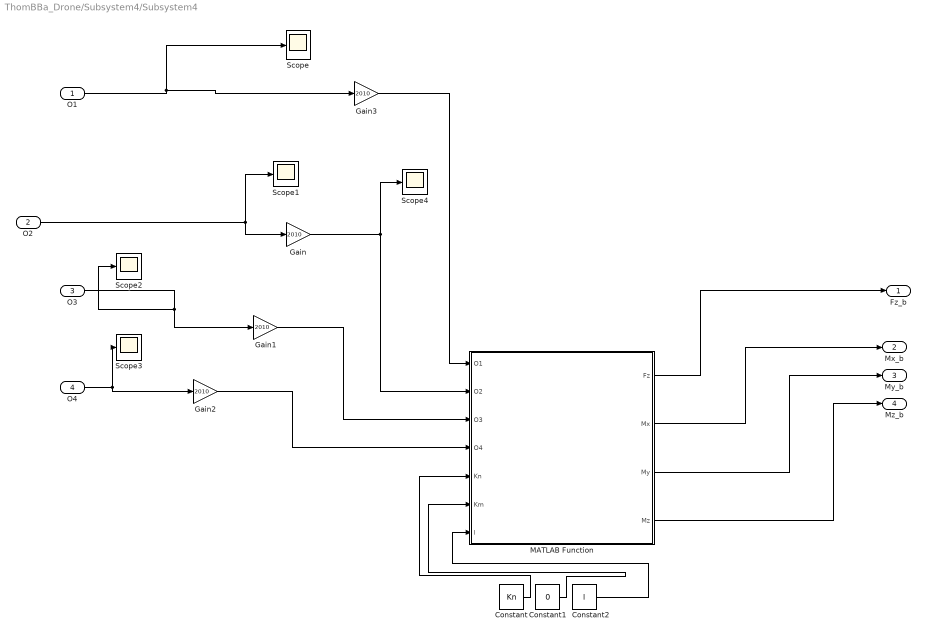
== system ThomBBa_Drone/Subsystem4/Subsystem4 ==
  O1 : Inport
  O2 : Inport  Port=2
  O3 : Inport  Port=3
  O4 : Inport  Port=4
  Constant : Constant  Value=Kn
  Constant1 : Constant  Value=0
  Constant2 : Constant  Value=l
  Gain{,1..3} (4 alike) : Gain  Gain=2010
  MATLAB Function : MATLAB Function  TreatAsAtomicUnit=on
  Scope{,1..4} (5 alike) : Scope
  Fz_b : Outport
  Mx_b : Outport  Port=2
  My_b : Outport  Port=3
  Mz_b : Outport  Port=4
  wires:
  MATLAB Function/1(Fz) -> Fz_b/1
  MATLAB Function/3(My) -> My_b/1
  MATLAB Function/4(Mz) -> Mz_b/1
  MATLAB Function/2(Mx) -> Mx_b/1
  Constant/1 -> MATLAB Function/5(Kn)
  Constant1/1 -> MATLAB Function/6(Km)
  Constant2/1 -> MATLAB Function/7(l)
  O2/1 -> Gain/1, Scope1/1
  Gain/1 -> Scope4/1, MATLAB Function/2(O2)
  O3/1 -> Gain1/1, Scope2/1
  Gain1/1 -> MATLAB Function/3(O3)
  O4/1 -> Gain2/1, Scope3/1
  Gain2/1 -> MATLAB Function/4(O4)
  O1/1 -> Gain3/1, Scope/1
  Gain3/1 -> MATLAB Function/1(O1)

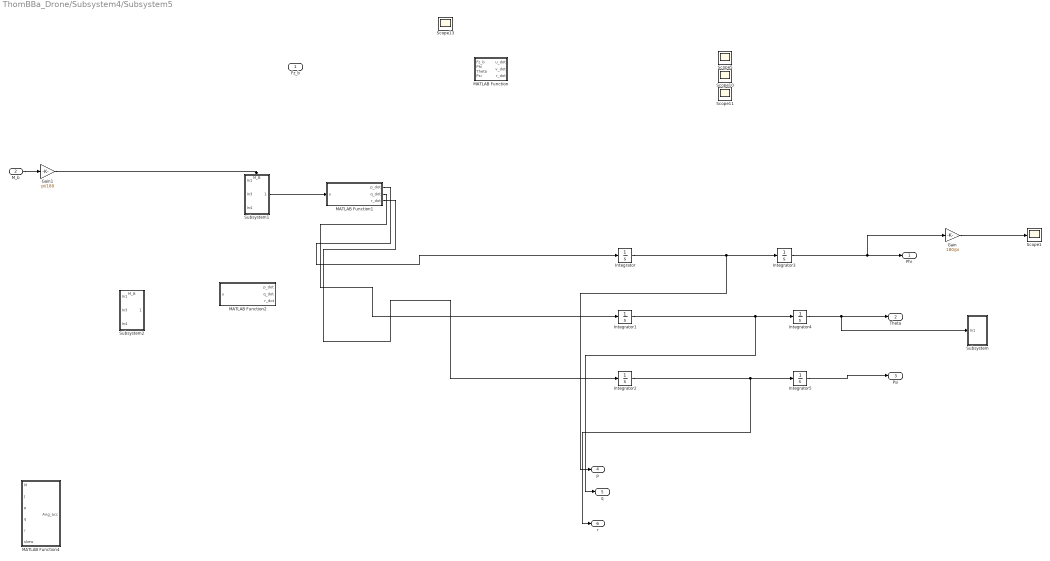
== system ThomBBa_Drone/Subsystem4/Subsystem5 ==
  Fz_b : Inport
  M_b : Inport  Port=2
  Gain : Gain  Gain=180/pi
  Gain1 : Gain  Gain=pi/180
  Integrator{,1..5} (6 alike) : Integrator
  MATLAB Function : MATLAB Function  TreatAsAtomicUnit=on
  MATLAB Function1 : MATLAB Function  TreatAsAtomicUnit=on
  MATLAB Function2 : MATLAB Function  TreatAsAtomicUnit=on
  MATLAB Function4 : MATLAB Function  TreatAsAtomicUnit=on
  Scope{1,5,10..11,13} (5 alike) : Scope
  Subsystem : Subsystem
  Subsystem1 : Subsystem
      settings: PortSchema="{\"entries\":[{\"content\":{\"sides\":[{\"content\":{\"connectorIds\":[\"In1\",\"In2\",\"In3\"]},\"type\":\"ConnectorPlacement.EquallySpacedRectSide\",\"uuid\":\"7e47c556-e7ea-4b92-bd73-2618c8afdf66\"},{\"content\":{\"connectorIds\":[\"Out1\"],\"side\":\"RIGHT\"},\"type\":\"ConnectorPlacement.EquallySpacedRectSide\",\"uuid\":\"8df0990a-ca25-4c34-ba36-930149f0a751\"},{\"content\":{\"connectorIds\":[\"In4\"],\"side\":\"TOP\"},\"type\":\"ConnectorPlacement.EquallySpacedRectSide\",\"uuid\":\"95f61e22-0c49-4373-add7-f41402ac3268\"},{\"content\":{\"side\":\"BOTTOM\"},\"type\":\"ConnectorPlacement.EquallySpacedRectSide\",\"uuid\":\"d89dd497-fba1-4e7c-8f58-49be8a5c83fa\"}]},\"type\":\"ConnectorPlacement.EquallySpacedConnector\",\"uuid\":\"f38f0594-1519-401a-85c8-093cd101747f\"}],\"packageUris\":[\"http://schema.mathworks.com/mf0/Connector/R2020b\"],\"version\":\"1.0\"}"
  Subsystem2 : Subsystem
      settings: PortSchema="{\"entries\":[{\"content\":{\"sides\":[{\"content\":{\"connectorIds\":[\"In1\",\"In2\",\"In3\"]},\"type\":\"ConnectorPlacement.EquallySpacedRectSide\",\"uuid\":\"7e47c556-e7ea-4b92-bd73-2618c8afdf66\"},{\"content\":{\"connectorIds\":[\"Out1\"],\"side\":\"RIGHT\"},\"type\":\"ConnectorPlacement.EquallySpacedRectSide\",\"uuid\":\"8df0990a-ca25-4c34-ba36-930149f0a751\"},{\"content\":{\"connectorIds\":[\"In4\"],\"side\":\"TOP\"},\"type\":\"ConnectorPlacement.EquallySpacedRectSide\",\"uuid\":\"95f61e22-0c49-4373-add7-f41402ac3268\"},{\"content\":{\"side\":\"BOTTOM\"},\"type\":\"ConnectorPlacement.EquallySpacedRectSide\",\"uuid\":\"d89dd497-fba1-4e7c-8f58-49be8a5c83fa\"}]},\"type\":\"ConnectorPlacement.EquallySpacedConnector\",\"uuid\":\"f38f0594-1519-401a-85c8-093cd101747f\"}],\"packageUris\":[\"http://schema.mathworks.com/mf0/Connector/R2020b\"],\"version\":\"1.0\"}"
  Phi : Outport
  Theta : Outport  Port=2
  Psi : Outport  Port=3
  p : Outport  Port=4
  q : Outport  Port=5
  r : Outport  Port=6
  wires:
  MATLAB Function1/1(p_dot) -> Integrator/1
  M_b/1 -> Gain1/1
  Integrator2/1 -> r/1, Integrator5/1
  Integrator/1 -> p/1, Integrator3/1
  Integrator1/1 -> q/1, Integrator4/1
  MATLAB Function1/2(q_dot) -> Integrator1/1
  MATLAB Function1/3(r_dot) -> Integrator2/1
  Gain/1 -> Scope1/1
  Integrator3/1 -> Gain/1, Phi/1
  Integrator4/1 -> Subsystem/1(In1), Theta/1
  Integrator5/1 -> Psi/1
  Gain1/1 -> Subsystem1/4(M_B)
  Subsystem1/1(Ang_acc_B) -> MATLAB Function1/1(u)

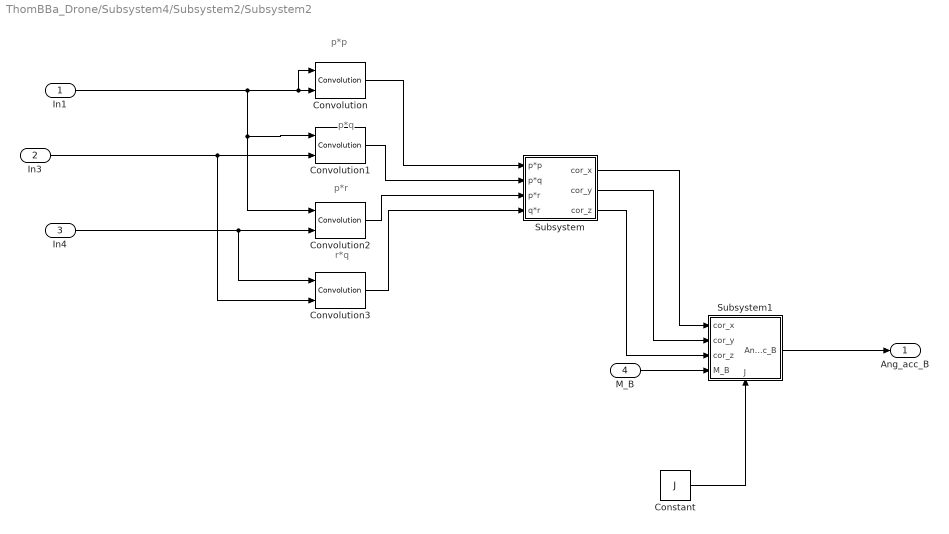
== system ThomBBa_Drone/Subsystem4/Subsystem2/Subsystem2 ==
  note: p*p
  note: p*q
  note: p*r
  note: r*q
  In1 : Inport
  In3 : Inport  Port=2
  In4 : Inport  Port=3
  M_B : Inport  Port=4
  Constant : Constant  Value=J
  Convolution{,1..3} (4 alike) : dspsigops/Convolution  domain=Time  roundingMode=Floor  overflowMode=off  outputDataTypeStr=Inherit: Same as accumulator  outputMin=[]  outputMax=[]  outputLastDataTypeStr=Inherit: Same as accumulator
  Subsystem : Subsystem
  Subsystem1 : Subsystem
      settings: PortSchema="{\"entries\":[{\"content\":{\"sides\":[{\"content\":{\"connectorIds\":[\"In1\",\"In2\",\"In3\",\"In4\"]},\"type\":\"ConnectorPlacement.EquallySpacedRectSide\",\"uuid\":\"7e47c556-e7ea-4b92-bd73-2618c8afdf66\"},{\"content\":{\"connectorIds\":[\"Out1\"],\"side\":\"RIGHT\"},\"type\":\"ConnectorPlacement.EquallySpacedRectSide\",\"uuid\":\"8df0990a-ca25-4c34-ba36-930149f0a751\"},{\"content\":{\"side\":\"TOP\"},\"type\":\"ConnectorPlacement.EquallySpacedRectSide\",\"uuid\":\"95f61e22-0c49-4373-add7-f41402ac3268\"},{\"content\":{\"connectorIds\":[\"In5\"],\"side\":\"BOTTOM\"},\"type\":\"ConnectorPlacement.EquallySpacedRectSide\",\"uuid\":\"ec23f56b-c0e0-46e7-a449-9b1d7a72ecb8\"}]},\"type\":\"ConnectorPlacement.EquallySpacedConnector\",\"uuid\":\"f38f0594-1519-401a-85c8-093cd101747f\"}],\"packageUris\":[\"http://schema.mathworks.com/mf0/Connector/R2020b\"],\"version\":\"1.0\"}"
  Ang_acc_B : Outport
  wires:
  Subsystem1/1(Ang_acc_B) -> Ang_acc_B/1
  Constant/1 -> Subsystem1/5(J)
  M_B/1 -> Subsystem1/4(M_B)
  Subsystem/3(cor_z) -> Subsystem1/3(cor_z)
  Subsystem/2(cor_y) -> Subsystem1/2(cor_y)
  Subsystem/1(cor_x) -> Subsystem1/1(cor_x)
  Convolution/1 -> Subsystem/1(p*p)
  Convolution1/1 -> Subsystem/2(p*q)
  Convolution2/1 -> Subsystem/3(p*r)
  Convolution3/1 -> Subsystem/4(q*r)
  In1/1 -> Convolution2/1, Convolution1/1, Convolution/1, Convolution/2
  In3/1 -> Convolution1/2, Convolution3/2
  In4/1 -> Convolution2/2, Convolution3/1

== system ThomBBa_Drone/Subsystem4/Subsystem5/Subsystem ==
  In1 : Inport
  Data Type Conversion : DataTypeConversion  SaturateOnIntegerOverflow=off  RndMeth=Floor
  Scope6 : Scope
  wires:
  In1/1 -> Scope6/1

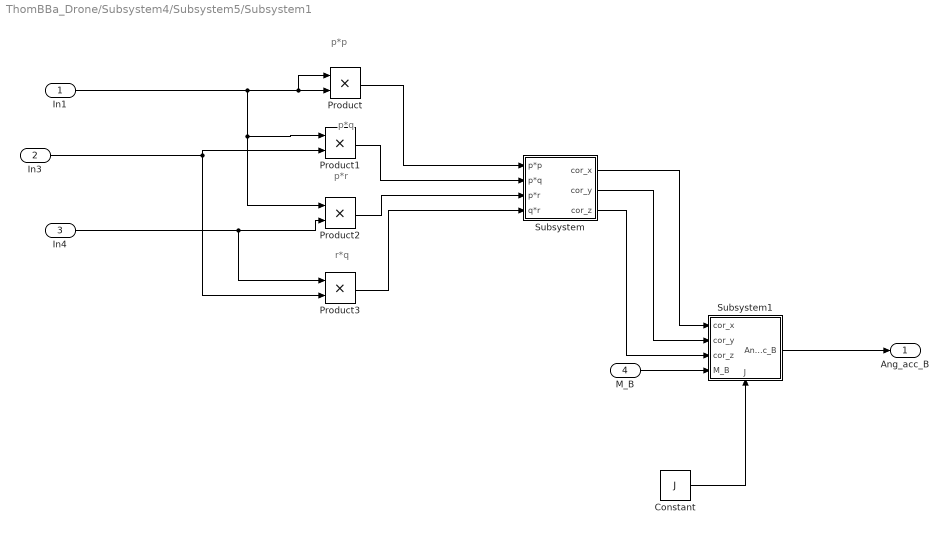
== system ThomBBa_Drone/Subsystem4/Subsystem5/Subsystem1 ==
  note: p*p
  note: p*q
  note: p*r
  note: r*q
  In1 : Inport
  In3 : Inport  Port=2
  In4 : Inport  Port=3
  M_B : Inport  Port=4
  Constant : Constant  Value=J
  Product{,1..3} (4 alike) : Product
  Subsystem : Subsystem
  Subsystem1 : Subsystem
      settings: PortSchema="{\"entries\":[{\"content\":{\"sides\":[{\"content\":{\"connectorIds\":[\"In1\",\"In2\",\"In3\",\"In4\"]},\"type\":\"ConnectorPlacement.EquallySpacedRectSide\",\"uuid\":\"7e47c556-e7ea-4b92-bd73-2618c8afdf66\"},{\"content\":{\"connectorIds\":[\"Out1\"],\"side\":\"RIGHT\"},\"type\":\"ConnectorPlacement.EquallySpacedRectSide\",\"uuid\":\"8df0990a-ca25-4c34-ba36-930149f0a751\"},{\"content\":{\"side\":\"TOP\"},\"type\":\"ConnectorPlacement.EquallySpacedRectSide\",\"uuid\":\"95f61e22-0c49-4373-add7-f41402ac3268\"},{\"content\":{\"connectorIds\":[\"In5\"],\"side\":\"BOTTOM\"},\"type\":\"ConnectorPlacement.EquallySpacedRectSide\",\"uuid\":\"ec23f56b-c0e0-46e7-a449-9b1d7a72ecb8\"}]},\"type\":\"ConnectorPlacement.EquallySpacedConnector\",\"uuid\":\"f38f0594-1519-401a-85c8-093cd101747f\"}],\"packageUris\":[\"http://schema.mathworks.com/mf0/Connector/R2020b\"],\"version\":\"1.0\"}"
  Ang_acc_B : Outport
  wires:
  Subsystem1/1(Ang_acc_B) -> Ang_acc_B/1
  Constant/1 -> Subsystem1/5(J)
  M_B/1 -> Subsystem1/4(M_B)
  Subsystem/3(cor_z) -> Subsystem1/3(cor_z)
  Subsystem/2(cor_y) -> Subsystem1/2(cor_y)
  Subsystem/1(cor_x) -> Subsystem1/1(cor_x)
  Product/1 -> Subsystem/1(p*p)
  Product1/1 -> Subsystem/2(p*q)
  Product2/1 -> Subsystem/3(p*r)
  Product3/1 -> Subsystem/4(q*r)
  In1/1 -> Product2/1, Product1/1, Product/2, Product/1
  In3/1 -> Product3/2, Product1/2
  In4/1 -> Product3/1, Product2/2

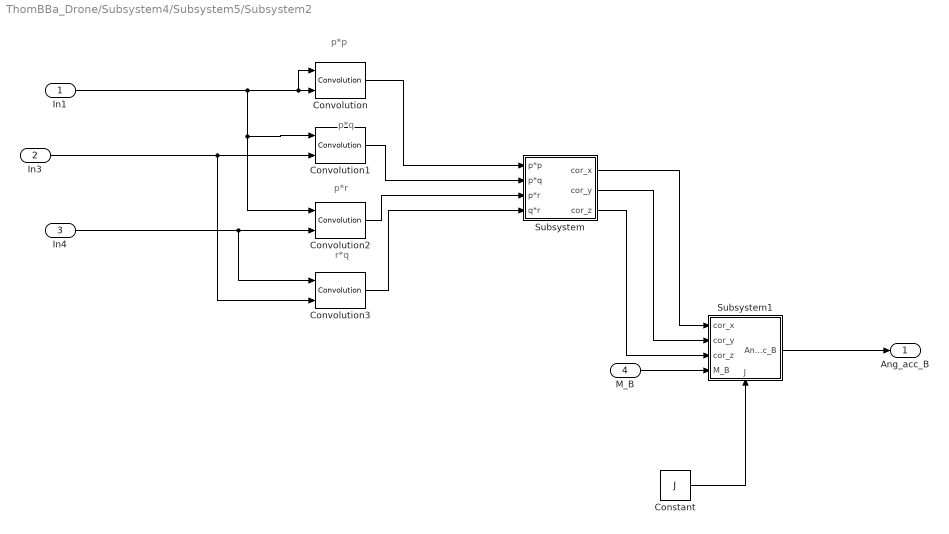
== system ThomBBa_Drone/Subsystem4/Subsystem5/Subsystem2 ==
  note: p*p
  note: p*q
  note: p*r
  note: r*q
  In1 : Inport
  In3 : Inport  Port=2
  In4 : Inport  Port=3
  M_B : Inport  Port=4
  Constant : Constant  Value=J
  Convolution{,1..3} (4 alike) : dspsigops/Convolution  domain=Time  roundingMode=Floor  overflowMode=off  outputDataTypeStr=Inherit: Same as accumulator  outputMin=[]  outputMax=[]  outputLastDataTypeStr=Inherit: Same as accumulator
  Subsystem : Subsystem
  Subsystem1 : Subsystem
      settings: PortSchema="{\"entries\":[{\"content\":{\"sides\":[{\"content\":{\"connectorIds\":[\"In1\",\"In2\",\"In3\",\"In4\"]},\"type\":\"ConnectorPlacement.EquallySpacedRectSide\",\"uuid\":\"7e47c556-e7ea-4b92-bd73-2618c8afdf66\"},{\"content\":{\"connectorIds\":[\"Out1\"],\"side\":\"RIGHT\"},\"type\":\"ConnectorPlacement.EquallySpacedRectSide\",\"uuid\":\"8df0990a-ca25-4c34-ba36-930149f0a751\"},{\"content\":{\"side\":\"TOP\"},\"type\":\"ConnectorPlacement.EquallySpacedRectSide\",\"uuid\":\"95f61e22-0c49-4373-add7-f41402ac3268\"},{\"content\":{\"connectorIds\":[\"In5\"],\"side\":\"BOTTOM\"},\"type\":\"ConnectorPlacement.EquallySpacedRectSide\",\"uuid\":\"ec23f56b-c0e0-46e7-a449-9b1d7a72ecb8\"}]},\"type\":\"ConnectorPlacement.EquallySpacedConnector\",\"uuid\":\"f38f0594-1519-401a-85c8-093cd101747f\"}],\"packageUris\":[\"http://schema.mathworks.com/mf0/Connector/R2020b\"],\"version\":\"1.0\"}"
  Ang_acc_B : Outport
  wires:
  Subsystem1/1(Ang_acc_B) -> Ang_acc_B/1
  Constant/1 -> Subsystem1/5(J)
  M_B/1 -> Subsystem1/4(M_B)
  Subsystem/3(cor_z) -> Subsystem1/3(cor_z)
  Subsystem/2(cor_y) -> Subsystem1/2(cor_y)
  Subsystem/1(cor_x) -> Subsystem1/1(cor_x)
  Convolution/1 -> Subsystem/1(p*p)
  Convolution1/1 -> Subsystem/2(p*q)
  Convolution2/1 -> Subsystem/3(p*r)
  Convolution3/1 -> Subsystem/4(q*r)
  In1/1 -> Convolution2/1, Convolution1/1, Convolution/1, Convolution/2
  In3/1 -> Convolution1/2, Convolution3/2
  In4/1 -> Convolution2/2, Convolution3/1

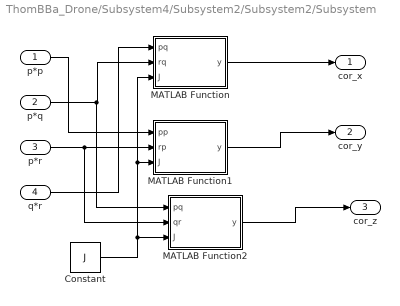
== system ThomBBa_Drone/Subsystem4/Subsystem2/Subsystem2/Subsystem ==
  p*p : Inport
  p*q : Inport  Port=2
  p*r : Inport  Port=3
  q*r : Inport  Port=4
  Constant : Constant  Value=J
  MATLAB Function : MATLAB Function  TreatAsAtomicUnit=on
  MATLAB Function1 : MATLAB Function  TreatAsAtomicUnit=on
  MATLAB Function2 : MATLAB Function  TreatAsAtomicUnit=on
  cor_x : Outport
  cor_y : Outport  Port=2
  cor_z : Outport  Port=3
  wires:
  MATLAB Function2/1(y) -> cor_z/1
  Constant/1 -> MATLAB Function2/3(J), MATLAB Function1/3(J), MATLAB Function/3(J)
  p*r/1 -> MATLAB Function1/2(rp), MATLAB Function2/2(qr)
  p*p/1 -> MATLAB Function1/1(pp)
  MATLAB Function1/1(y) -> cor_y/1
  p*q/1 -> MATLAB Function/2(rq), MATLAB Function2/1(pq)
  q*r/1 -> MATLAB Function/1(pq)
  MATLAB Function/1(y) -> cor_x/1

== system ThomBBa_Drone/Subsystem4/Subsystem2/Subsystem2/Subsystem1 ==
  cor_x : Inport
  cor_y : Inport  Port=2
  cor_z : Inport  Port=3
  M_B : Inport  Port=4
  J : Inport  Port=5
  MATLAB Function : MATLAB Function  TreatAsAtomicUnit=on
  Ang_acc_B : Outport
  wires:
  MATLAB Function/1(Ang_acc_B) -> Ang_acc_B/1
  J/1 -> MATLAB Function/5(J)
  M_B/1 -> MATLAB Function/4(M_B)
  cor_x/1 -> MATLAB Function/1(cor_x)
  cor_z/1 -> MATLAB Function/3(cor_z)
  cor_y/1 -> MATLAB Function/2(cor_y)

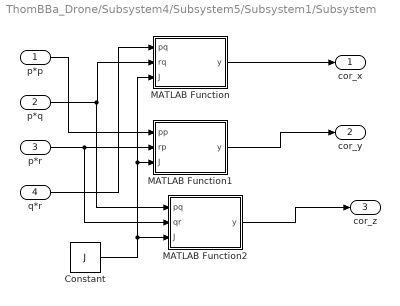
== system ThomBBa_Drone/Subsystem4/Subsystem5/Subsystem1/Subsystem ==
  p*p : Inport
  p*q : Inport  Port=2
  p*r : Inport  Port=3
  q*r : Inport  Port=4
  Constant : Constant  Value=J
  MATLAB Function : MATLAB Function  TreatAsAtomicUnit=on
  MATLAB Function1 : MATLAB Function  TreatAsAtomicUnit=on
  MATLAB Function2 : MATLAB Function  TreatAsAtomicUnit=on
  cor_x : Outport
  cor_y : Outport  Port=2
  cor_z : Outport  Port=3
  wires:
  MATLAB Function2/1(y) -> cor_z/1
  Constant/1 -> MATLAB Function2/3(J), MATLAB Function1/3(J), MATLAB Function/3(J)
  p*r/1 -> MATLAB Function1/2(rp), MATLAB Function2/2(qr)
  p*p/1 -> MATLAB Function1/1(pp)
  MATLAB Function1/1(y) -> cor_y/1
  p*q/1 -> MATLAB Function/2(rq), MATLAB Function2/1(pq)
  q*r/1 -> MATLAB Function/1(pq)
  MATLAB Function/1(y) -> cor_x/1

== system ThomBBa_Drone/Subsystem4/Subsystem5/Subsystem1/Subsystem1 ==
  cor_x : Inport
  cor_y : Inport  Port=2
  cor_z : Inport  Port=3
  M_B : Inport  Port=4
  J : Inport  Port=5
  MATLAB Function : MATLAB Function  TreatAsAtomicUnit=on
  Ang_acc_B : Outport
  wires:
  MATLAB Function/1(Ang_acc_B) -> Ang_acc_B/1
  J/1 -> MATLAB Function/5(J)
  M_B/1 -> MATLAB Function/4(M_B)
  cor_x/1 -> MATLAB Function/1(cor_x)
  cor_z/1 -> MATLAB Function/3(cor_z)
  cor_y/1 -> MATLAB Function/2(cor_y)

== system ThomBBa_Drone/Subsystem4/Subsystem5/Subsystem2/Subsystem ==
  p*p : Inport
  p*q : Inport  Port=2
  p*r : Inport  Port=3
  q*r : Inport  Port=4
  Constant : Constant  Value=J
  MATLAB Function : MATLAB Function  TreatAsAtomicUnit=on
  MATLAB Function1 : MATLAB Function  TreatAsAtomicUnit=on
  MATLAB Function2 : MATLAB Function  TreatAsAtomicUnit=on
  cor_x : Outport
  cor_y : Outport  Port=2
  cor_z : Outport  Port=3
  wires:
  MATLAB Function2/1(y) -> cor_z/1
  Constant/1 -> MATLAB Function2/3(J), MATLAB Function1/3(J), MATLAB Function/3(J)
  p*r/1 -> MATLAB Function1/2(rp), MATLAB Function2/2(qr)
  p*p/1 -> MATLAB Function1/1(pp)
  MATLAB Function1/1(y) -> cor_y/1
  p*q/1 -> MATLAB Function/2(rq), MATLAB Function2/1(pq)
  q*r/1 -> MATLAB Function/1(pq)
  MATLAB Function/1(y) -> cor_x/1

== system ThomBBa_Drone/Subsystem4/Subsystem5/Subsystem2/Subsystem1 ==
  cor_x : Inport
  cor_y : Inport  Port=2
  cor_z : Inport  Port=3
  M_B : Inport  Port=4
  J : Inport  Port=5
  MATLAB Function : MATLAB Function  TreatAsAtomicUnit=on
  Ang_acc_B : Outport
  wires:
  MATLAB Function/1(Ang_acc_B) -> Ang_acc_B/1
  J/1 -> MATLAB Function/5(J)
  M_B/1 -> MATLAB Function/4(M_B)
  cor_x/1 -> MATLAB Function/1(cor_x)
  cor_z/1 -> MATLAB Function/3(cor_z)
  cor_y/1 -> MATLAB Function/2(cor_y)

== matlab function ThomBBa_Drone/Subsystem4/Subsystem2/MATLAB Function4 ==
  data: M input; Ang_acc output; J input; p input; q input; r input; skew input

function Ang_acc  = Ang_A_B(M,J,p, q, r, skew)







Ang_acc = inv(J)*(M-skew*(J*[p;q;r]));

end

== matlab function ThomBBa_Drone/MATLAB Function ==
  data: Phi input; y output; Theta input; Th input
function y = fcn(Phi, Theta, Th)

y = Th + 0.01*Th*((abs((sin(Phi))*abs((1+sin(Theta)))+abs((sin(Theta))*abs((1+sin(Phi)))))));

== matlab function ThomBBa_Drone/Subsystem4/Subsystem2/MATLAB Function6 ==
  data: u input; p_dot output; q_dot output; r_dot output; Phi input; Theta input
function [p_dot,q_dot,r_dot] = Rot(u,Phi,Theta)



p_dot =  [1 sin(Phi)*tan(Theta)   cos(Phi)*tan(Theta)]*u;
q_dot =  [  0        cos(Phi)            -sin(Phi)]*u    ;
r_dot =  [ 0  sin(Phi)*sec(Theta)   cos(Phi)*sec(Theta)]*u;


 



end

== matlab function ThomBBa_Drone/MATLAB Function1 ==
  data: Phi input; y output; Theta input; Th input
function y = fcn(Phi, Theta, Th)

y = Th + 0.01*Th*((abs((sin(Phi))*abs((1+sin(Theta)))+abs((sin(Theta))*abs((1+sin(Phi)))))));

== matlab function ThomBBa_Drone/Subsystem4/Subsystem2/MATLAB Function2 ==
  data: x_air_damping_ratio input; z_air_damping_ratio input; u input; Phi input; u_air_damping output; Theta input
function u_air_damping = fcn(x_air_damping_ratio, z_air_damping_ratio, u,Phi, Theta)

u_air_damping = (abs(z_air_damping_ratio*sin(Theta))+x_air_damping_ratio*cos(Phi))*u;

== matlab function ThomBBa_Drone/Subsystem4/Subsystem5/MATLAB Function4 ==
  data: M input; Ang_acc output; J input; p input; q input; r input; skew input

function Ang_acc  = Ang_A_B(M,J,p, q, r, skew)







Ang_acc = inv(J)*(M-skew*(J*[p;q;r]));

end

== matlab function ThomBBa_Drone/Subsystem4/Subsystem2/Subsystem2/Subsystem/MATLAB Function ==
  data: pq input; rq input; y output; J input
function y = fcn(pq, rq,J)

y = rq*(J(3,3)-J(2,2))-pq*(J(1,3));
end

== matlab function ThomBBa_Drone/Subsystem4/Subsystem5/Subsystem1/Subsystem/MATLAB Function ==
  data: pq input; rq input; y output; J input
function y = fcn(pq, rq,J)

y = rq*(J(3,3)-J(2,2))-pq*(J(1,3));
end

== matlab function ThomBBa_Drone/Subsystem4/Subsystem5/Subsystem1/Subsystem/MATLAB Function1 ==
  data: pp input; rp input; y output; J input
function y = fcn(pp,rp, J)

y = rp*(J(1,1)-J(3,3))-pp*(J(1,3));
end

== matlab function ThomBBa_Drone/Subsystem4/Subsystem5/Subsystem1/Subsystem/MATLAB Function2 ==
  data: pq input; qr input; y output; J input
function y = fcn(pq,qr,J)

y = qr*(J(1,3))+pq*(J(2,2)-J(1,1));
end

== matlab function ThomBBa_Drone/Subsystem4/Subsystem5/Subsystem1/Subsystem1/MATLAB Function ==
  data: cor_x input; Ang_acc_B output; cor_y input; cor_z input; M_B input; J input
function Ang_acc_B = fcn(cor_x, cor_y, cor_z, M_B, J)

Ang_acc_B = inv(J)*(M_B - [cor_x;cor_y;cor_z]);
end

== matlab function ThomBBa_Drone/Subsystem4/Subsystem5/Subsystem2/Subsystem/MATLAB Function ==
  data: pq input; rq input; y output; J input
function y = fcn(pq, rq,J)

y = rq*(J(3,3)-J(2,2))-pq*(J(1,3));
end

== matlab function ThomBBa_Drone/Subsystem4/Subsystem5/Subsystem2/Subsystem/MATLAB Function1 ==
  data: pp input; rp input; y output; J input
function y = fcn(pp,rp, J)

y = rp*(J(1,1)-J(3,3))-pp*(J(1,3));
end

== matlab function ThomBBa_Drone/Subsystem4/Subsystem5/Subsystem2/Subsystem/MATLAB Function2 ==
  data: pq input; qr input; y output; J input
function y = fcn(pq,qr,J)

y = qr*(J(1,3))+pq*(J(2,2)-J(1,1));
end
